simulink model "vRTHS_ASMC"  (R2019a)
settings: Solver=ode4  StartTime=0.0  StopTime=tend  FixedStep=dt_rths  RelTol=1e-3  EnableMultiTasking=on
values from neighbouring files (symbols this model uses):
  a2 = 4.23e6    (= 4230000)    [Actuator_id.m]
  a3 = [3.3-uncer*1.3,3.3+uncer*1.3]    [Actuator_id.m]
  compd = [dt_rths 1]    [F2_controller.m]
  compn = [2*dt_rths 1]    [F2_controller.m]
  d1 = 53354    [F2_controller.m]
  d2 = 0.00010595    [F2_controller.m]
  d3 = 0.021072    [F2_controller.m]
  dt_rths = 1/fs    (= 0.000244140625)    [Elcentro_results.m]    (also in Main_ANSMC.m; Main_PI.m)
  E_sw = 1    [Elcentro_results.m]
  eq_intensity = .4    (= 0.4)    [Elcentro_results.m]    (also in Main_ANSMC.m; Main_PI.m)
  k0 = 1000000    [Elcentro_results.m]    (also in Main_ANSMC.m)
  Para = [alpha_hat0 alpha_bar lambda lambda1 eta sw]    [F2_controller.m]
  Psi_hat0 = (alpha_hat0-[z1,z2])'    [Elcentro_results.m]    (also in Main_ANSMC.m)
  Rx = rms_noise_DT/dt_rths    [F2_controller.m]
  theta0 = 0.1    [Elcentro_results.m]    (also in Main_ANSMC.m)
  xinitial = zeros(2,1)    [F2_controller.m]
  z1 = 1600    [Elcentro_results.m]    (also in Main_ANSMC.m)
  z2 = 2    [Elcentro_results.m]    (also in Main_ANSMC.m)
undefined symbols (not defined in the file or in its folder): a1_beta0, A_ns, B_ns, beta1, beta2, C_ns, CE, Continuous, D_ns, Gsnsr_DT, Gsnsr_FT, KE, ME, Seed_snr, tend, Time
libraries: simulink x3, ctrlSharedLib x1, sldrtlib x1
settings Model: Creator=IISL_0175  LastModifiedBy=hongwei
settings DataIOCC: SaveFormat=StructureWithTime  ReturnWorkspaceOutputs=off
settings OptimizationCC: LifeSpan=inf
settings DebuggingCC: InheritedTsInSrcMsg=none  SFUnexpectedBacktrackingDiag=warning  SFNoUnconditionalDefaultTransitionDiag=warning  SFExecutionAtInitializationDiag=none  ArithmeticOperatorsInVariantConditions=warning
settings HardwareCC: ProdBitPerSizeT=32  ProdBitPerPtrDiffT=32  ProdWordSize=32  ProdHWDeviceType=Specified
settings SFSimCC: SimUseLocalCustomCode=off
settings RTWCC: RTWUseLocalCustomCode=off
settings CodeAppCC: StateflowObjectComments=on
settings GRTTargetCC: TargetLangStandard=C89/C90 (ANSI)  GeneratePreprocessorConditionals=Disable all
settings ConfigComp: CovMetricSettings=dw  CovHtmlReporting=on  CovSaveCumulativeToWorkspaceVar=on  CovSaveSingleToWorkspaceVar=on  CovExternalEMLEnable=off

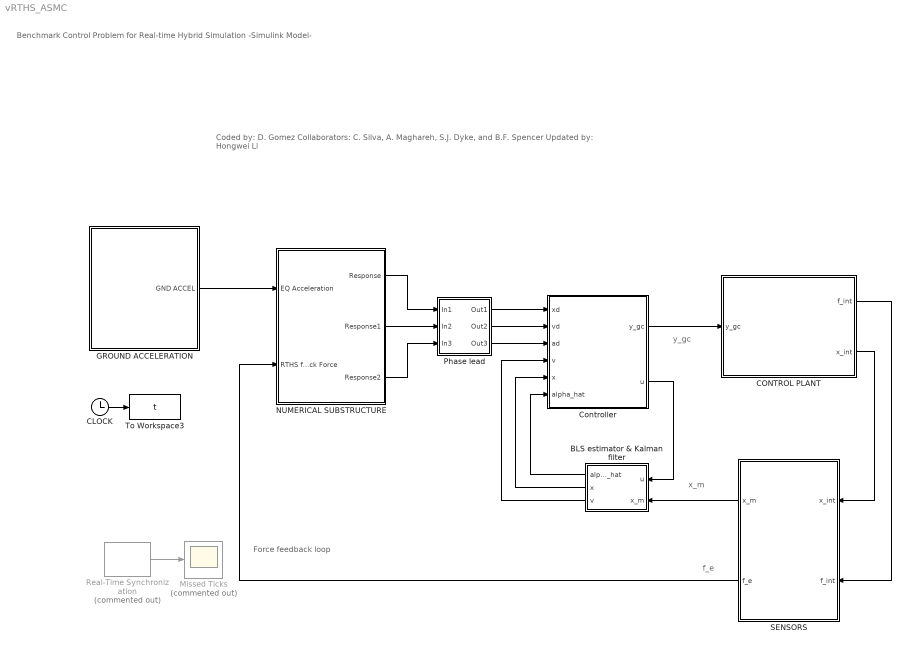
== system vRTHS_ASMC ==
  note: Force
      | feedback loop
  note: Benchmark Control Problem for Real-time Hybrid Simulation
      | -Simulink Model-
  note: Coded by: D. Gomez
      | Collaborators: C. Silva, A. Maghareh, S.J. Dyke, and B.F. Spencer
      | Updated by: Hongwei Li
  note: y_gc
  note: f_e
  note: x_m
  BLS estimator & Kalman filter : Subsystem
  CLOCK : Clock
  CONTROL PLANT : Subsystem
      mask Display: image(imread('PlantSW2.PNG'));
  Controller : Subsystem
  GROUND ACCELERATION : Subsystem
  Missed Ticks : Scope  Commented=on
  NUMERICAL SUBSTRUCTURE : Subsystem
      mask Display: image(imread('Num_sub.png'));
  Phase lead : Subsystem
  Real-Time Synchronization : sldrtlib/Real-Time Synchronization  Commented=on  SampleTime=dt_rths  MaxMissedTicks=10000  ShowMissedTicks=on  YieldWhenWaiting=off
  SENSORS : Subsystem
  To Workspace3 : ToWorkspace  VariableName=t  SampleTime=-1
  wires:
  CLOCK/1 -> To Workspace3/1
  CONTROL PLANT/2(x_int) -> SENSORS/1(x_int)
  Controller/1(y_gc) -> CONTROL PLANT/1(y_gc)
  Real-Time Synchronization/1 -> Missed Ticks/1
  SENSORS/1(x_m) -> BLS estimator & Kalman filter/2(x_m)
  GROUND ACCELERATION/1(GND ACCEL) -> NUMERICAL SUBSTRUCTURE/1(EQ Acceleration)
  CONTROL PLANT/1(f_int) -> SENSORS/2(f_int)
  SENSORS/2("f_e ") -> NUMERICAL SUBSTRUCTURE/2(RTHS feedback Force)
  NUMERICAL SUBSTRUCTURE/1(Response) -> Phase lead/1(In1)
  Phase lead/1(Out1) -> Controller/1(xd)
  Phase lead/2(Out2) -> Controller/2(vd)
  Phase lead/3(Out3) -> Controller/3(ad)
  NUMERICAL SUBSTRUCTURE/2(Response1) -> Phase lead/2(In2)
  NUMERICAL SUBSTRUCTURE/3(Response2) -> Phase lead/3(In3)
  Controller/2(u) -> BLS estimator & Kalman filter/1(u)
  BLS estimator & Kalman filter/1(alpha_hat) -> Controller/6(alpha_hat)
  BLS estimator & Kalman filter/2(x) -> Controller/5(x)
  BLS estimator & Kalman filter/3(v) -> Controller/4(v)

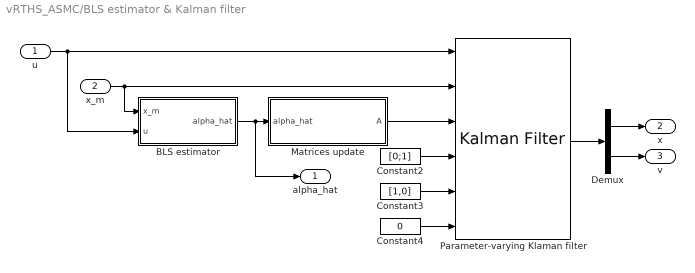
== system vRTHS_ASMC/BLS estimator & Kalman filter ==
  u : Inport
  x_m : Inport  Port=2
  BLS estimator : Subsystem
  Constant2 : Constant  Value=[0;1]  VectorParams1D=off
  Constant3 : Constant  Value=[1,0]  VectorParams1D=off
  Constant4 : Constant  Value=0  VectorParams1D=off
  Demux : Demux  Outputs=2
  Matrices update : MATLAB Function  TreatAsAtomicUnit=on
  Parameter-varying Klaman filter : ctrlSharedLib/Kalman Filter  TimeDomain=Continuous-Time  UseCurrentEstimator=on  ModelSource=Input port  ModelSourceVariable=ss(0.95,1,1,0,1)  A=0.95  B=1  C=1  D=0  NumberOfStates=2  NumberOfInputs=1  NumberOfOutputs=1  InitialEstimateSource=Dialog  X0=xinitial  P0=1e-10  UseK=off  UseGH=off  NumberOfProcessNoiseInputs=1  G=1  TimeInvariantG=on  H=0  TimeInvariantH=on  Q=0  TimeInvariantQ=on  R=Rx  TimeInvariantR=on  N=0  TimeInvariantN=on  AddInputPort=on  AddEnablePort=off  OutputEstimatedY=off  OutputP=off  Ts=-1
      settings: SourceProductBaseCode=CT
  alpha_hat : Outport
  x : Outport  Port=2
  v : Outport  Port=3
  wires:
  BLS estimator/1(alpha_hat) -> alpha_hat/1, Matrices update/1(alpha_hat)
  Matrices update/1(A) -> Parameter-varying Klaman filter/3
  Constant2/1 -> Parameter-varying Klaman filter/4
  Constant3/1 -> Parameter-varying Klaman filter/5
  Constant4/1 -> Parameter-varying Klaman filter/6
  Parameter-varying Klaman filter/1 -> Demux/1
  Demux/1 -> x/1
  Demux/2 -> v/1
  x_m/1 -> BLS estimator/1(x_m), Parameter-varying Klaman filter/2
  u/1 -> BLS estimator/2(u), Parameter-varying Klaman filter/1

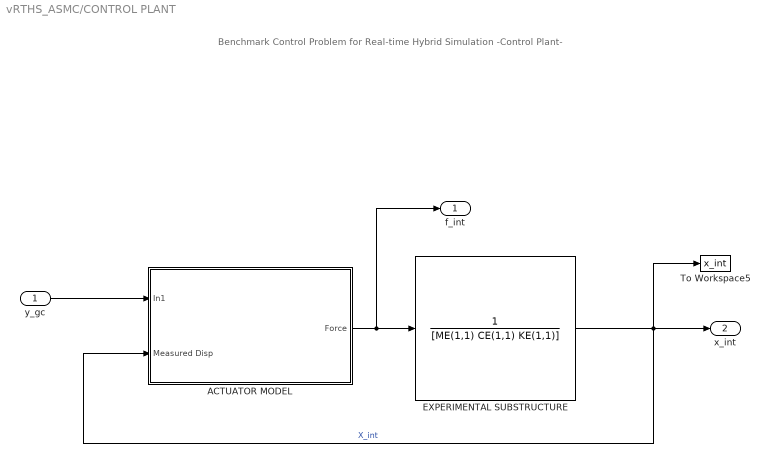
== system vRTHS_ASMC/CONTROL PLANT ==
  note: Benchmark Control Problem for Real-time Hybrid Simulation
      | -Control Plant-
  y_gc : Inport
  ACTUATOR MODEL : Subsystem
      mask Display: image(imread('ActuatorSW2.PNG'));
  EXPERIMENTAL SUBSTRUCTURE : TransferFcn  Numerator=1  Denominator=[ME(1,1) CE(1,1) KE(1,1)]
      mask Display: image(imread('ESSW2.PNG'));
  To Workspace5 : ToWorkspace  VariableName=x_int  SampleTime=-1
  f_int : Outport
  x_int : Outport  Port=2
  wires:
  EXPERIMENTAL SUBSTRUCTURE/1 -> ACTUATOR MODEL/2(Measured Disp), To Workspace5/1, x_int/1  "X_int"
  ACTUATOR MODEL/1(Force) -> f_int/1, EXPERIMENTAL SUBSTRUCTURE/1
  y_gc/1 -> ACTUATOR MODEL/1(In1)

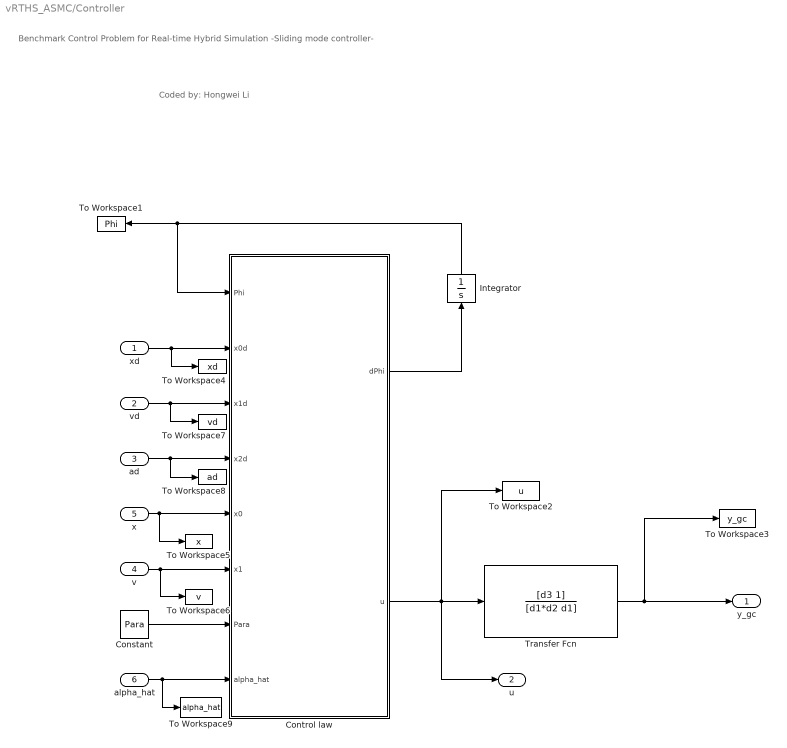
== system vRTHS_ASMC/Controller ==
  note: Coded by: Hongwei Li
  note: Benchmark Control Problem for Real-time Hybrid Simulation
      | -Sliding mode controller-
  xd : Inport
  vd : Inport  Port=2
  ad : Inport  Port=3
  v : Inport  Port=4
  x : Inport  Port=5
  alpha_hat : Inport  Port=6
  Constant : Constant  Value=Para  VectorParams1D=off
  Control law : MATLAB Function  TreatAsAtomicUnit=on
  Integrator : Integrator
  To Workspace1 : ToWorkspace  VariableName=Phi  SampleTime=-1
  To Workspace2 : ToWorkspace  VariableName=u  SampleTime=-1
  To Workspace3 : ToWorkspace  VariableName=y_gc  SampleTime=-1
  To Workspace4 : ToWorkspace  VariableName=xd  SampleTime=-1
  To Workspace5 : ToWorkspace  VariableName=x  SampleTime=-1
  To Workspace6 : ToWorkspace  VariableName=v  SampleTime=-1
  To Workspace7 : ToWorkspace  VariableName=vd  SampleTime=-1
  To Workspace8 : ToWorkspace  VariableName=ad  SampleTime=-1
  To Workspace9 : ToWorkspace  VariableName=alpha_hat  SampleTime=-1
  Transfer Fcn : TransferFcn  Numerator=[d3 1]  Denominator=[d1*d2 d1]
  y_gc : Outport
  u : Outport  Port=2
  wires:
  ad/1 -> To Workspace8/1, Control law/4(x2d)
  vd/1 -> To Workspace7/1, Control law/3(x1d)
  x/1 -> To Workspace5/1, Control law/5(x0)
  Constant/1 -> Control law/7(Para)
  Integrator/1 -> To Workspace1/1, Control law/1(Phi)
  v/1 -> To Workspace6/1, Control law/6(x1)
  xd/1 -> To Workspace4/1, Control law/2(x0d)
  Control law/1(dPhi) -> Integrator/1
  Transfer Fcn/1 -> y_gc/1, To Workspace3/1
  Control law/2(u) -> u/1, To Workspace2/1, Transfer Fcn/1
  alpha_hat/1 -> To Workspace9/1, Control law/8(alpha_hat)

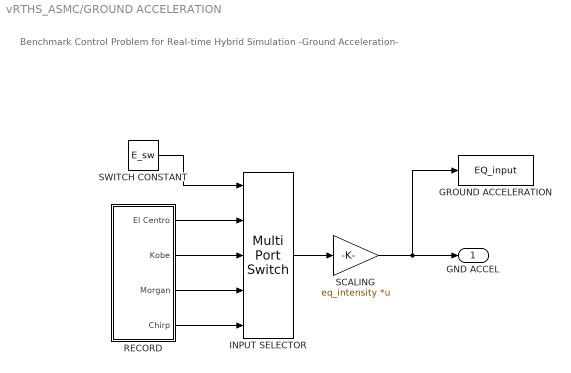
== system vRTHS_ASMC/GROUND ACCELERATION ==
  note: Benchmark Control Problem for Real-time Hybrid Simulation
      | -Ground Acceleration-
  GROUND ACCELERATION : ToWorkspace  VariableName=EQ_input  SampleTime=-1
  INPUT SELECTOR : MultiPortSwitch  Inputs=4
  "RECORD " : Subsystem
  SCALING : Gain  Gain=eq_intensity  Multiplication=Matrix(K*u)
  SWITCH CONSTANT : Constant  Value=E_sw
  GND ACCEL : Outport
  wires:
  INPUT SELECTOR/1 -> SCALING/1
  SWITCH CONSTANT/1 -> INPUT SELECTOR/1
  "RECORD "/1(El Centro) -> INPUT SELECTOR/2
  "RECORD "/2(Kobe) -> INPUT SELECTOR/3
  "RECORD "/3(Morgan) -> INPUT SELECTOR/4
  SCALING/1 -> GROUND ACCELERATION/1, GND ACCEL/1
  "RECORD "/4(Chirp) -> INPUT SELECTOR/5

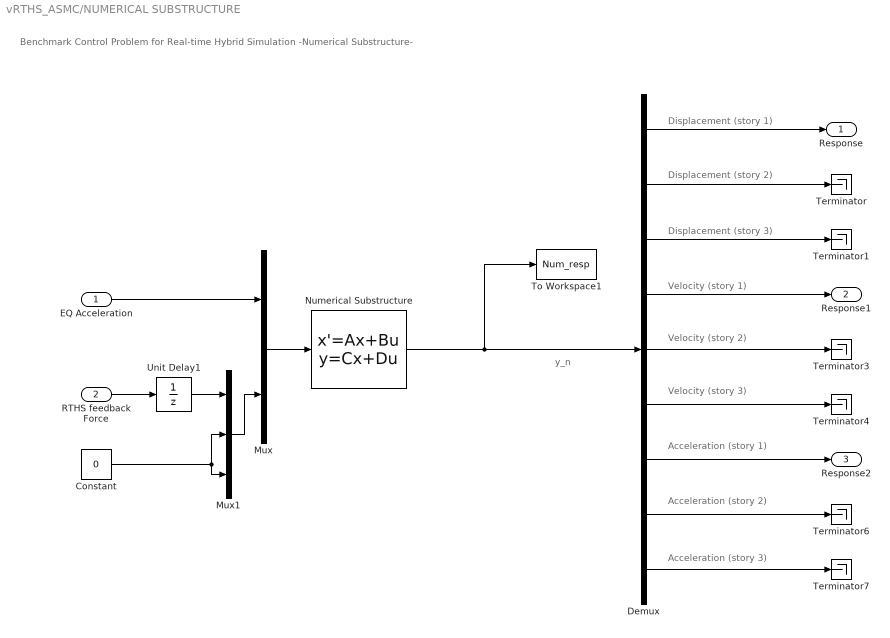
== system vRTHS_ASMC/NUMERICAL SUBSTRUCTURE ==
  note: y_n
  note: Benchmark Control Problem for Real-time Hybrid Simulation
      | -Numerical Substructure-
  note: Velocity (story 3)
  note: Displacement (story 3)
  note: Displacement (story 1)
  note: Acceleration (story 1)
  note: Velocity (story 1)
  note: Velocity (story 2)
  note: Acceleration (story 3)
  note: Displacement (story 2)
  note: Acceleration (story 2)
  EQ Acceleration : Inport
  RTHS feedback Force : Inport  Port=2
  Constant : Constant  Value=0
  Demux : Demux  Outputs=9
  Mux : Mux  Inputs=2
  Mux1 : Mux  Inputs=3
  Numerical Substructure : StateSpace  A=A_ns  B=B_ns  C=C_ns  D=D_ns  InitialCondition=0
  Terminator{,1,3..4,6..7} (6 alike) : Terminator
  To Workspace1 : ToWorkspace  VariableName=Num_resp  SaveFormat=Timeseries  SampleTime=-1
  Unit Delay1 : UnitDelay  SampleTime=-1  HasFrameUpgradeWarning=on
  Response : Outport
  Response1 : Outport  Port=2
  Response2 : Outport  Port=3
  wires:
  Mux/1 -> Numerical Substructure/1
  EQ Acceleration/1 -> Mux/1
  RTHS feedback Force/1 -> Unit Delay1/1
  Numerical Substructure/1 -> To Workspace1/1, Demux/1
  Demux/2 -> Terminator/1
  Demux/7 -> Response2/1
  Demux/8 -> Terminator6/1
  Demux/9 -> Terminator7/1
  Demux/4 -> Response1/1
  Demux/6 -> Terminator4/1
  Demux/5 -> Terminator3/1
  Demux/1 -> Response/1
  Demux/3 -> Terminator1/1
  Constant/1 -> Mux1/2, Mux1/3
  Mux1/1 -> Mux/2
  Unit Delay1/1 -> Mux1/1

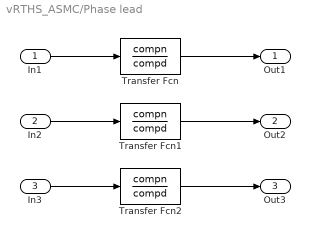
== system vRTHS_ASMC/Phase lead ==
  In1 : Inport
  In2 : Inport  Port=2
  In3 : Inport  Port=3
  Transfer Fcn : TransferFcn  Numerator=compn  Denominator=compd
  Transfer Fcn1 : TransferFcn  Numerator=compn  Denominator=compd
  Transfer Fcn2 : TransferFcn  Numerator=compn  Denominator=compd
  Out1 : Outport
  Out2 : Outport  Port=2
  Out3 : Outport  Port=3
  wires:
  In1/1 -> Transfer Fcn/1
  Transfer Fcn/1 -> Out1/1
  In2/1 -> Transfer Fcn1/1
  Transfer Fcn1/1 -> Out2/1
  In3/1 -> Transfer Fcn2/1
  Transfer Fcn2/1 -> Out3/1

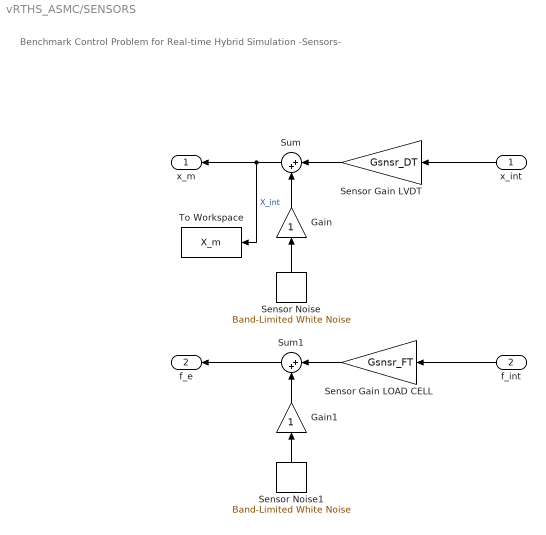
== system vRTHS_ASMC/SENSORS ==
  note: Benchmark Control Problem for Real-time Hybrid Simulation
      | -Sensors-
  x_int : Inport
  f_int : Inport  Port=2
  Gain : Gain
  Gain1 : Gain
  Sensor Noise : simulink/Sources/Band-Limited White Noise  Cov=rms_noise_DT  Ts=dt_rths  seed=double(Seed_snr.Seed)
  Sensor Noise1 : simulink/Sources/Band-Limited White Noise  Cov=rms_noise_FT  Ts=dt_rths  seed=double(Seed_snr.Seed)
  Sensor Gain LVDT : Gain  Gain=Gsnsr_DT  SaturateOnIntegerOverflow=on  OutDataTypeStr=Inherit: Same as input  ParamDataTypeStr=Inherit: Same as input
  Sensor Gain LOAD CELL : Gain  Gain=Gsnsr_FT  SaturateOnIntegerOverflow=on  OutDataTypeStr=Inherit: Same as input  ParamDataTypeStr=Inherit: Same as input
  Sum : Sum  Inputs=|++  SaturateOnIntegerOverflow=on  InputSameDT=on  OutDataTypeStr=Inherit: Same as first input
  Sum1 : Sum  Inputs=|++  SaturateOnIntegerOverflow=on  InputSameDT=on  OutDataTypeStr=Inherit: Same as first input
  To Workspace : ToWorkspace  VariableName=X_m  SaveFormat=Timeseries  SampleTime=-1
  x_m : Outport
  "f_e " : Outport  Port=2
  wires:
  Sensor Gain LVDT/1 -> Sum/1
  Sensor Noise/1 -> Gain/1
  x_int/1 -> Sensor Gain LVDT/1
  Sensor Gain LOAD CELL/1 -> Sum1/1
  Sum1/1 -> "f_e "/1
  Sensor Noise1/1 -> Gain1/1
  f_int/1 -> Sensor Gain LOAD CELL/1
  Sum/1 -> x_m/1, To Workspace/1  "X_int"
  Gain/1 -> Sum/2
  Gain1/1 -> Sum1/2

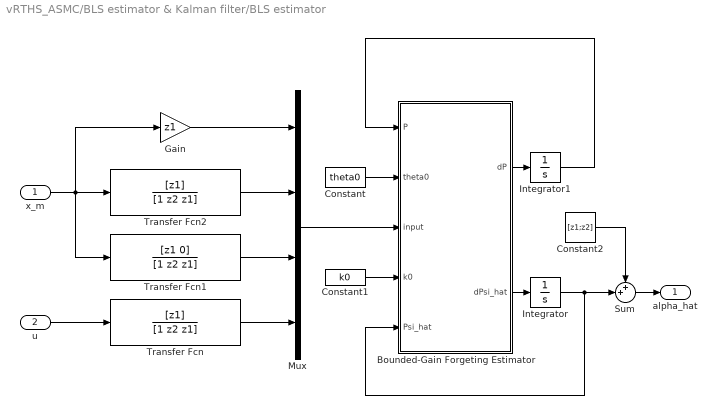
== system vRTHS_ASMC/BLS estimator & Kalman filter/BLS estimator ==
  x_m : Inport
  u : Inport  Port=2
  Bounded-Gain Forgeting Estimator : MATLAB Function  TreatAsAtomicUnit=on
  Constant : Constant  Value=theta0
  Constant1 : Constant  Value=k0
  Constant2 : Constant  Value=[z1;z2]  VectorParams1D=off
  Gain : Gain  Gain=z1
  Integrator : Integrator  InitialCondition=Psi_hat0
  Integrator1 : Integrator  InitialCondition=k0*eye(2)
  Mux : Mux
  Sum : Sum  Inputs=++|
  Transfer Fcn : TransferFcn  Numerator=[z1]  Denominator=[1 z2 z1]
  Transfer Fcn1 : TransferFcn  Numerator=[z1 0]  Denominator=[1 z2 z1]
  Transfer Fcn2 : TransferFcn  Numerator=[z1]  Denominator=[1 z2 z1]
  alpha_hat : Outport
  wires:
  Bounded-Gain Forgeting Estimator/2(dPsi_hat) -> Integrator/1
  Integrator/1 -> Sum/2, Bounded-Gain Forgeting Estimator/5(Psi_hat)
  Integrator1/1 -> Bounded-Gain Forgeting Estimator/1(P)
  Constant1/1 -> Bounded-Gain Forgeting Estimator/4(k0)
  Constant/1 -> Bounded-Gain Forgeting Estimator/2(theta0)
  Bounded-Gain Forgeting Estimator/1(dP) -> Integrator1/1
  x_m/1 -> Transfer Fcn1/1, Gain/1, Transfer Fcn2/1
  u/1 -> Transfer Fcn/1
  Gain/1 -> Mux/1
  Transfer Fcn2/1 -> Mux/2
  Transfer Fcn1/1 -> Mux/3
  Transfer Fcn/1 -> Mux/4
  Mux/1 -> Bounded-Gain Forgeting Estimator/3(input)
  Sum/1 -> alpha_hat/1
  Constant2/1 -> Sum/1

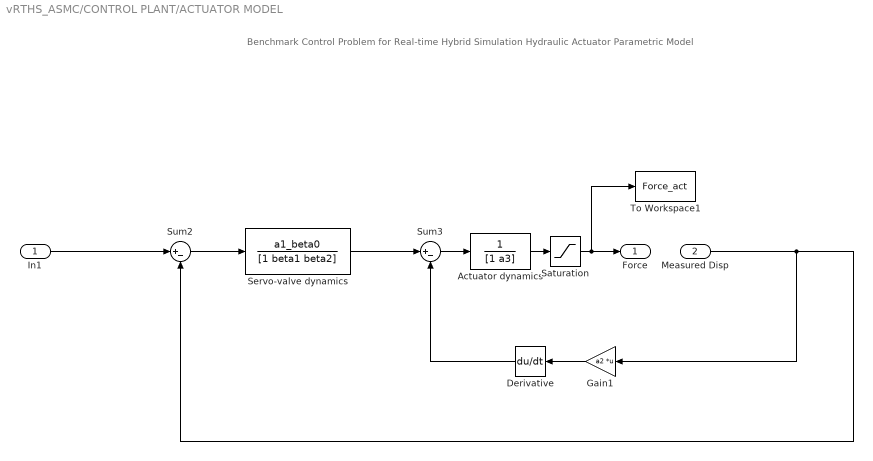
== system vRTHS_ASMC/CONTROL PLANT/ACTUATOR MODEL ==
  note: Benchmark Control Problem for Real-time Hybrid Simulation
      | Hydraulic Actuator Parametric Model
  In1 : Inport
  Measured Disp : Inport  Port=2
  Actuator dynamics : TransferFcn  Numerator=1  Denominator=[1 a3]
  Derivative : Derivative
  Gain1 : Gain  Gain=a2  Multiplication=Matrix(K*u)
  Saturation : Saturate  UpperLimit=8900  LowerLimit=-8900
  Servo-valve dynamics : TransferFcn  Numerator=a1_beta0  Denominator=[1 beta1 beta2]
  Sum2 : Sum  Inputs=|+-
  Sum3 : Sum  Inputs=|+-
  To Workspace1 : ToWorkspace  VariableName=Force_act  SampleTime=-1
  Force : Outport
  wires:
  In1/1 -> Sum2/1
  Actuator dynamics/1 -> Saturation/1
  Servo-valve dynamics/1 -> Sum3/1
  Sum2/1 -> Servo-valve dynamics/1
  Gain1/1 -> Derivative/1
  Derivative/1 -> Sum3/2
  Sum3/1 -> Actuator dynamics/1
  Measured Disp/1 -> Sum2/2, Gain1/1
  Saturation/1 -> To Workspace1/1, Force/1

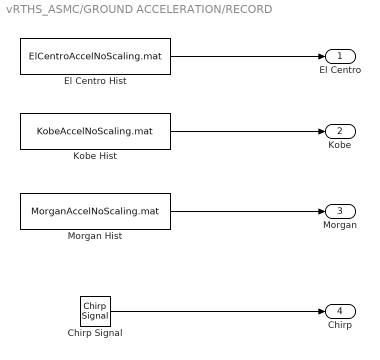
== system vRTHS_ASMC/GROUND ACCELERATION/RECORD  ==
  Chirp Signal : simulink/Sources/Chirp Signal  f1=f_ini  T=tend  f2=f_end
  El Centro Hist : FromFile  FileName=ElCentroAccelNoScaling.mat
  Kobe Hist : FromFile  FileName=KobeAccelNoScaling.mat
  Morgan Hist : FromFile  FileName=MorganAccelNoScaling.mat
  El Centro : Outport
  Kobe : Outport  Port=2
  Morgan : Outport  Port=3
  Chirp : Outport  Port=4
  wires:
  Morgan Hist/1 -> Morgan/1
  Kobe Hist/1 -> Kobe/1
  El Centro Hist/1 -> El Centro/1
  Chirp Signal/1 -> Chirp/1

== matlab function vRTHS_ASMC/BLS estimator & Kalman filter/BLS estimator/Bounded-Gain Forgeting Estimator ==
  data: P input; theta0 input; input input; k0 input; Psi_hat input; dP output; dPsi_hat output
function [dP,dPsi_hat] = BGFE(P,theta0,input,k0,Psi_hat)
y=input(1)-input(4);
W=-[input(2) input(3)];
yhat=W*Psi_hat;
e1=yhat-y;
dPsi_hat=-P*W'*e1;
theta=theta0*(1-norm(P)/k0);
dP=theta*P-P*(W'*W)*P;

== matlab function vRTHS_ASMC/BLS estimator & Kalman filter/Matrices update ==
  data: alpha_hat input; A output
function A  = Matrices(alpha_hat)
A=[0 1;-alpha_hat'];

== matlab function vRTHS_ASMC/Controller/Control law ==
  data: Phi input; x0d input; x1d input; x2d input; x0 input; x1 input; dPhi output; Para input; u output; alpha_hat input
function [dPhi,u]  = Controller(Phi,x0d,x1d,x2d,x0,x1,Para,alpha_hat)
a_bar=Para(3:4);
lambda=Para(5);
lambda1=Para(6);
eta=Para(7);
sw=Para(8);

f=[x0;x1];
e0=x0-x0d; e1=x1-x1d;
E=e1+lambda*e0;
h=x2d-lambda*e1;
u_hat=alpha_hat'*f+h;

k0=a_bar*abs(f);
if sw~=0
    k=lambda1*Phi;
    dPhi=eta+k0-k;
else
    k=k0+eta;
    dPhi=0;
end
if abs(E)>=Phi
    sat=sign(E);
else
    sat=E/Phi;
end
uc=-k*sat;
u=u_hat+uc;
